simulink model "aeropendulum_model"  (R2021b)
settings: Solver=FixedStepAuto  StartTime=0.0  StopTime=12  FixedStep=0.05  RelTol=1e-3
model workspace (MATLAB code in the model file):
  | % masa wahadla
  | m = 0.120; % [kg]
  | 
  | % przyspieszenie grawitacyjne
  | g = 9.81; % [m/s^2]
  | 
  | % tarcie wiskotyczne
  | % @ref https://koyo.jtekt.co.jp/en/support/bearing-knowledge/8-4000.html
  | c = 0.00700; % [Nms/rad]
  | 
  | % dlugosc wahadla
  | l = 0.25; % [m]
  | 
  | % moment bezwladnosci
  | J = m*l*l; % [kgm^2]
  | 
  | % odleglosc osi od srodka masy
  | d = 0.25; % [m]
  | 
  | % strefa martwa
  | deadzone = 500; % [rpm]
  | 
  | % charakterystyka smigla predkosc-ciag
  | p1_thrust = 0.5;
  | p1_krpm = 3.0;
  | p2_thrust = -0.4;
  | p2_krpm = 3.0;
  | dz = deadzone/1000;
  | p1 = polyfit([(-p1_krpm+dz) dz p1_krpm], [p1_thrust 0 p1_thrust], 2);
  | p2 = polyfit([-p2_krpm -dz (p2_krpm-dz)], [p2_thrust 0 p2_thrust], 2);
  | 
  | % wspolczynnik dla smigla w "zla" strone
  | % alfa_rev = 0.014; % [Ns/rad]
  | 
  | % wspolczynnik dla smigla w "dobra" strone
  | % alfa = 0.019 % [Ns/rad]
  | 
settings Model: Creator=adria  LastModifiedBy=adria

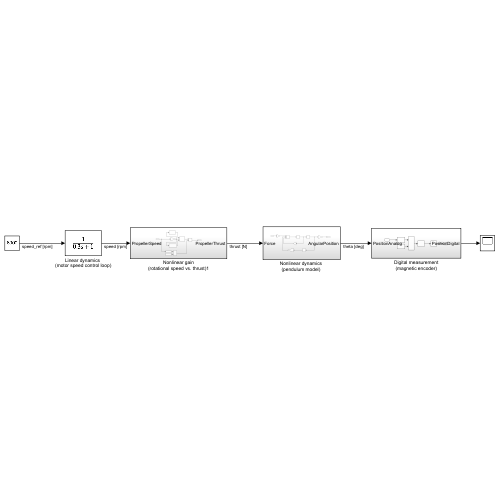
[thumbnail: Simulink's stored preview of the top-level diagram]
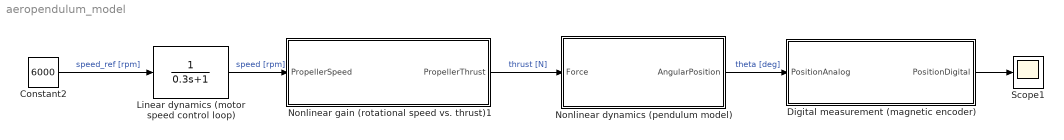
== system aeropendulum_model ==
  Constant2 : Constant  Value=6000
  Digital measurement (magnetic encoder) : Subsystem
  Linear dynamics (motor speed control loop) : TransferFcn  Denominator=[0.3 1]
  "Nonlinear dynamics (pendulum model) " : Subsystem
  Nonlinear gain (rotational speed vs. thrust)1 : Subsystem
  Scope1 : Scope
  wires:
  Digital measurement (magnetic encoder)/1(PositionDigital) -> Scope1/1
  "Nonlinear dynamics (pendulum model) "/1(AngularPosition) -> Digital measurement (magnetic encoder)/1(PositionAnalog)  "theta [deg]"
  Constant2/1 -> Linear dynamics (motor speed control loop)/1  "speed_ref [rpm]"
  Nonlinear gain (rotational speed vs. thrust)1/1(PropellerThrust) -> "Nonlinear dynamics (pendulum model) "/1(Force)  "thrust [N]"
  Linear dynamics (motor speed control loop)/1 -> Nonlinear gain (rotational speed vs. thrust)1/1(PropellerSpeed)  "speed [rpm]"

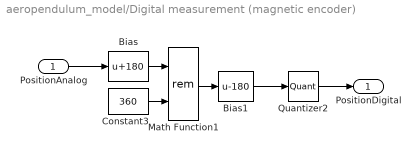
== system aeropendulum_model/Digital measurement (magnetic encoder) ==
  PositionAnalog : Inport
  Bias : Bias  Bias=180
  Bias1 : Bias  Bias=-180
  Constant3 : Constant  Value=360
  Math Function1 : Math  Operator=rem  SaturateOnIntegerOverflow=on
  Quantizer2 : Quantizer  QuantizationInterval=(360 - 360/4096)/4096
  PositionDigital : Outport
  wires:
  Bias1/1 -> Quantizer2/1
  Math Function1/1 -> Bias1/1
  Bias/1 -> Math Function1/1
  PositionAnalog/1 -> Bias/1
  Constant3/1 -> Math Function1/2
  Quantizer2/1 -> PositionDigital/1

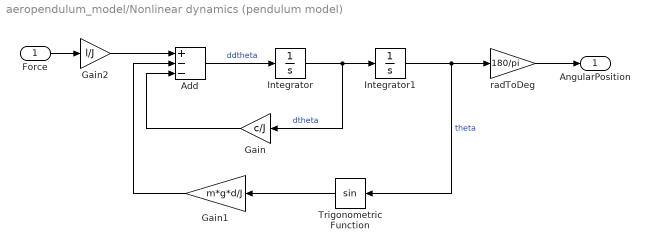
== system aeropendulum_model/Nonlinear dynamics (pendulum model)  ==
  Force : Inport
  Add : Sum  Inputs=+--
  Gain : Gain  Gain=c/J
  Gain1 : Gain  Gain=m*g*d/J
  Gain2 : Gain  Gain=l/J
  Integrator : Integrator
  Integrator1 : Integrator
  Trigonometric Function : Trigonometry
  radToDeg : Gain  Gain=180/pi
  AngularPosition : Outport
  wires:
  Trigonometric Function/1 -> Gain1/1
  Integrator1/1 -> Trigonometric Function/1, radToDeg/1  "theta"
  Gain/1 -> Add/3
  Gain2/1 -> Add/1
  Integrator/1 -> Gain/1, Integrator1/1  "dtheta"
  Force/1 -> Gain2/1
  radToDeg/1 -> AngularPosition/1
  Gain1/1 -> Add/2
  Add/1 -> Integrator/1  "ddtheta"

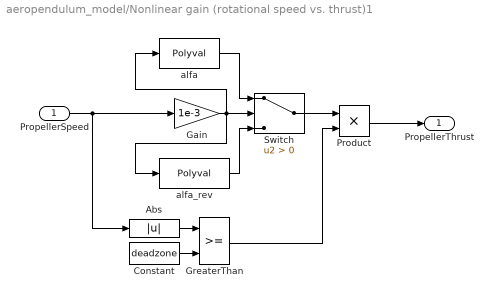
== system aeropendulum_model/Nonlinear gain (rotational speed vs. thrust)1 ==
  PropellerSpeed : Inport
  Abs : Abs
  Constant : Constant  Value=deadzone
  Gain : Gain  Gain=1e-3
  GreaterThan : RelationalOperator  OutDataTypeStr=boolean  RndMeth=Simplest
  Product : Product
  Switch : Switch  Criteria=u2 > Threshold
  alfa : Polyval  Coefs="[0.0400   -0.0200    0.0000]"
  alfa_rev : Polyval  Coefs="[-0.0267   -0.0133   -0.0000]"
  PropellerThrust : Outport
  wires:
  alfa/1 -> Switch/1
  alfa_rev/1 -> Switch/3
  Gain/1 -> alfa_rev/1, alfa/1, Switch/2
  Switch/1 -> Product/1
  Product/1 -> PropellerThrust/1
  PropellerSpeed/1 -> Abs/1, Gain/1
  Constant/1 -> GreaterThan/2
  Abs/1 -> GreaterThan/1
  GreaterThan/1 -> Product/2
